simulink model "fft_sysgen_double"  (R2014b)
settings: Solver=FixedStepDiscrete  SolverMode=SingleTasking  StartTime=0.0  StopTime=Ts*Ns*10  RelTol=1e-3
PreLoadFcn:
  | cd C:\Users\Tim-UML\Documents\GitHub\MA_1\FFT_sysgen_double
InitFcn:
  | cd C:\Users\Tim-UML\Documents\GitHub\MA_1\FFT_sysgen_double
StartFcn:
  | cd C:\Users\Tim-UML\Documents\GitHub\MA_1\FFT_sysgen_double
undefined symbols (not defined in the file or in its folder): Ns, Radix, Ts
libraries: xbsIndex_r4 x12, dspxfrm3 x1
settings Model: Creator=Tim-UML  LastModifiedBy=Tim-UML

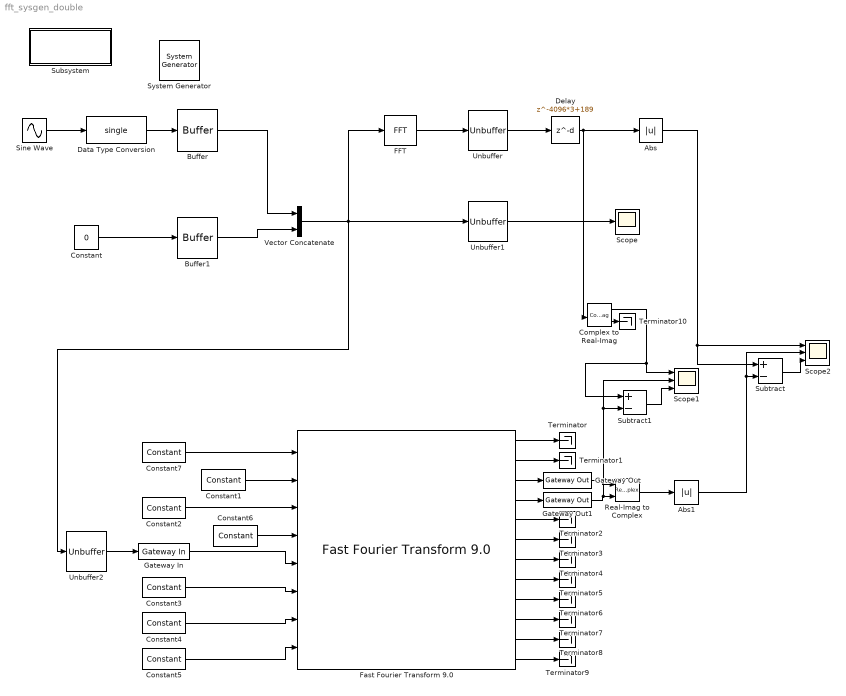
== system fft_sysgen_double ==
  " System Generator" : xbsIndex_r4/ System Generator  Tag=genX  xilinxfamily=zynq  part=xc7z020  speed=-1  package=clg400  synthesis_tool=Vivado  clock_wrapper=Clock Enables  directory=./netlist  proj_type=Vivado  Synth_file=Vivado Synthesis Defaults  Impl_file=Vivado Implementation Defaults  testbench=on  simulink_period=Ts/2  sysclk_period=10  dcm_input_clock_period=10  incr_netlist=off  trim_vbits=Everywhere in SubSystem  dbl_ovrd=According to Block Masks  core_generation=According to Block Masks  run_coregen=off  deprecated_control=off  eval_field=0  block_type=sysgen
  Abs : Abs
  Abs1 : Abs
  Buffer : Buffer  N=Ns  TreatMby1Signals=One channel
  Buffer1 : Buffer  N=Ns  TreatMby1Signals=One channel
  Complex to Real-Imag : ComplexToRealImag
  Constant : Constant  Value=0  OutDataTypeStr=single  SampleTime=Ts
  Constant1 : xbsIndex_r4/Constant  const=1  gui_display_data_type=Fixed-point  arith_type=Unsigned  n_bits=1  bin_pt=0  preci_type=Single  exp_width=8  frac_width=24  explicit_period=off  period=1  equ=P=C  opselect=C  inp2=PCIN>>17  opr=+  inp1=P  carry=CIN  dbl_ovrd=off  block_type=constant
  Constant2 : xbsIndex_r4/Constant  const=1  gui_display_data_type=Boolean  arith_type=Boolean  n_bits=16  bin_pt=14  preci_type=Single  exp_width=8  frac_width=24  explicit_period=off  period=1  equ=P=C  opselect=C  inp2=PCIN>>17  opr=+  inp1=P  carry=CIN  dbl_ovrd=off  block_type=constant
  Constant3 : xbsIndex_r4/Constant  const=1  gui_display_data_type=Boolean  arith_type=Boolean  n_bits=16  bin_pt=14  preci_type=Single  exp_width=8  frac_width=24  explicit_period=off  period=1  equ=P=C  opselect=C  inp2=PCIN>>17  opr=+  inp1=P  carry=CIN  dbl_ovrd=off  block_type=constant
  Constant4 : xbsIndex_r4/Constant  const=0  gui_display_data_type=Boolean  arith_type=Boolean  n_bits=16  bin_pt=14  preci_type=Single  exp_width=8  frac_width=24  explicit_period=off  period=1  equ=P=C  opselect=C  inp2=PCIN>>17  opr=+  inp1=P  carry=CIN  dbl_ovrd=off  block_type=constant
  Constant5 : xbsIndex_r4/Constant  const=1  gui_display_data_type=Boolean  arith_type=Boolean  n_bits=16  bin_pt=14  preci_type=Single  exp_width=8  frac_width=24  explicit_period=off  period=1  equ=P=C  opselect=C  inp2=PCIN>>17  opr=+  inp1=P  carry=CIN  dbl_ovrd=off  block_type=constant
  Constant6 : xbsIndex_r4/Constant  const=0  gui_display_data_type=Floating-point  arith_type=Floating-point  n_bits=16  bin_pt=14  preci_type=Single  exp_width=8  frac_width=24  explicit_period=off  period=1  equ=P=C  opselect=C  inp2=PCIN>>17  opr=+  inp1=P  carry=CIN  dbl_ovrd=off  block_type=constant
  Constant7 : xbsIndex_r4/Constant  const=0  gui_display_data_type=Fixed-point  arith_type=Unsigned  n_bits=12  bin_pt=0  preci_type=Single  exp_width=8  frac_width=24  explicit_period=off  period=1  equ=P=C  opselect=C  inp2=PCIN>>17  opr=+  inp1=P  carry=CIN  dbl_ovrd=off  block_type=constant
  Data Type Conversion : DataTypeConversion  OutDataTypeStr=single
  Delay : Delay  DelayLength=4096*3+189  InitialCondition=0
  FFT : dspxfrm3/FFT  CompMethod=Table lookup  TableOpt=NEW  TableOptActive=Speed  BitRevOrder=off  InheritFFTLength=on  FFTLength=64  WrapInput=on  RowConvenienceOn=on  FFTImplementation=Radix-2  SkipNorm=off  firstCoeffDataTypeStr=Inherit: Same word length as input  firstCoeffLastDataTypeStr=Inherit: Same word length as input  outputMin=[]  outputMax=[]  roundingMode=Floor  overflowMode=off
  "Fast Fourier Transform 9.0 " : xbsIndex_r4/Fast Fourier Transform 9.0   transform_length=4096  target_clock_frequency=250  target_data_throughput=50  implementation_options=pipelined_streaming_io  run_time_configurable_transform_length=off  phase_factor_width=25  scaling_options=scaled  rounding_modes=convergent_rounding  aclken=off  aresetn=off  cyclic_prefix_insertion=off  output_ordering=natural_order  throttle_scheme=nonrealtime  xk_index=off  ovflo=off  trim_axipin_name=on  memory_options_data=block_ram  memory_options_phase_factors=block_ram  number_of_stages_using_block_ram_for_data_and_phase_factors=3  memory_options_reorder=block_ram  memory_options_hybrid=off  complex_mult_type=use_mults_resources  butterfly_type=use_luts  channels=1  input_ordering=natural_order  input_width=16  ip_name=Fast Fourier Transform  ip_version=9.0  dsptool_ready=true  ipcore_usecache=true  ipcore_useipmodelcache=true  wrapper_available=true  port_translation_map={ 'aclken' => 'en', 'aresetn' => 'rst'}  data_format=fixed_point  block_type=xfft_v9_0
  Gateway In : xbsIndex_r4/Gateway In  gui_display_data_type=Floating-point  arith_type=Floating-point  n_bits=16  bin_pt=14  preci_type=Single  exp_width=8  frac_width=24  rows=1  columns=1  quantization="Round  (unbiased: +/- Inf)"  overflow=Saturate  period=Ts/2  UseAsADC=off  ADCChannel='1'  interface=None  automatic_assignment=on  address_offset=hex2dec('00')  intf_description=''  timing_constraint=None  locs_specified=off  LOCs={}  io_standard={}  inherit_from_input=off  hdl_port=on  dbl_ovrd=off  block_type=gatewayin
  Gateway Out : xbsIndex_r4/Gateway Out  inherit_from_input=on  hdl_port=on  rows=1  columns=1  UseAsDAC=off  DACChannel='1'  interface=None  automatic_assignment=on  address_offset=hex2dec('00')  intf_description=''  timing_constraint=None  locs_specified=off  LOCs={}  io_standard={}  block_type=gatewayout
  Gateway Out1 : xbsIndex_r4/Gateway Out  inherit_from_input=on  hdl_port=on  rows=1  columns=1  UseAsDAC=off  DACChannel='1'  interface=None  automatic_assignment=on  address_offset=hex2dec('00')  intf_description=''  timing_constraint=None  locs_specified=off  LOCs={}  io_standard={}  block_type=gatewayout
  Real-Imag to Complex : RealImagToComplex
  Scope : Scope
      settings: MaxDataPoints=15000
  Scope1 : Scope  NumInputPorts=3
      settings: YMin=-5~-5~-5  YMax=5~5~5
  Scope2 : Scope  NumInputPorts=3
      settings: YMin=-5~-5~-5  YMax=5~5~5  SaveName=ScopeData2
  Sine Wave : Sin  SineType=Sample based  SampleTime=Ts
  Subsystem : Subsystem  mask(Model Parameters){SampleTime=20e-9, SampleCount=2048}
      mask prompts: SampleTime "Sample Time [s]"; SampleCount "Sample Count"
      mask init:
      | initScript_fft_sysgen_double
      mask Display: disp('Edit Model\n Parameters')
  Subtract : Sum  Inputs=+-
  Subtract1 : Sum  Inputs=+-
  Terminator{,1..10} (11 alike) : Terminator
  Unbuffer : Unbuffer  SampleBasedProcessing=Same as frame based
  Unbuffer1 : Unbuffer  SampleBasedProcessing=Same as frame based
  Unbuffer2 : Unbuffer  SampleBasedProcessing=Same as frame based
  Vector Concatenate : Concatenate  Mode=Multidimensional array
  wires:
  Sine Wave/1 -> Data Type Conversion/1
  Buffer/1 -> Vector Concatenate/1
  FFT/1 -> Unbuffer/1
  Constant/1 -> Buffer1/1
  Buffer1/1 -> Vector Concatenate/2
  Vector Concatenate/1 -> Unbuffer2/1, FFT/1, Unbuffer1/1
  Unbuffer1/1 -> Scope/1
  Unbuffer/1 -> Delay/1
  Constant1/1 -> "Fast Fourier Transform 9.0 "/2
  Constant2/1 -> "Fast Fourier Transform 9.0 "/3
  Constant3/1 -> "Fast Fourier Transform 9.0 "/6
  Constant4/1 -> "Fast Fourier Transform 9.0 "/7
  Constant5/1 -> "Fast Fourier Transform 9.0 "/8
  Gateway In/1 -> "Fast Fourier Transform 9.0 "/5
  Constant6/1 -> "Fast Fourier Transform 9.0 "/4
  Unbuffer2/1 -> Gateway In/1
  "Fast Fourier Transform 9.0 "/1 -> Terminator/1
  "Fast Fourier Transform 9.0 "/2 -> Terminator1/1
  "Fast Fourier Transform 9.0 "/5 -> Terminator2/1
  "Fast Fourier Transform 9.0 "/6 -> Terminator3/1
  "Fast Fourier Transform 9.0 "/7 -> Terminator4/1
  "Fast Fourier Transform 9.0 "/8 -> Terminator5/1
  "Fast Fourier Transform 9.0 "/9 -> Terminator6/1
  "Fast Fourier Transform 9.0 "/10 -> Terminator7/1
  "Fast Fourier Transform 9.0 "/11 -> Terminator8/1
  "Fast Fourier Transform 9.0 "/12 -> Terminator9/1
  "Fast Fourier Transform 9.0 "/3 -> Gateway Out/1
  "Fast Fourier Transform 9.0 "/4 -> Gateway Out1/1
  Gateway Out/1 -> Real-Imag to Complex/1
  Real-Imag to Complex/1 -> Abs1/1
  Abs1/1 -> Subtract/2, Scope2/2
  Subtract/1 -> Scope2/3
  Constant7/1 -> "Fast Fourier Transform 9.0 "/1
  Data Type Conversion/1 -> Buffer/1
  Abs/1 -> Subtract/1, Scope2/1
  Gateway Out1/1 -> Scope1/2, Subtract1/2, Real-Imag to Complex/2
  Subtract1/1 -> Scope1/3
  Complex to Real-Imag/1 -> Scope1/1, Subtract1/1
  Complex to Real-Imag/2 -> Terminator10/1
  Delay/1 -> Complex to Real-Imag/1, Abs/1

== system fft_sysgen_double/Subsystem ==
